simulink model "Hybrid_PV_Wind_System"  (R2018a)
settings: Solver=ode3  StartTime=0.0  StopTime=80  FixedStep=1e-4  RelTol=1e-3  EnableMultiTasking=on
InitFcn:
  | clear all ;
  | clc;
  | 
  | %%Wind System%%
  | 
  | %wind speed
  | Z_data=10;
  | Z_hub=85;
  | Z_0=0.03;
  | 
  | %Turbine
  | R_=45;
  | G=100;
  | lambda_opt=7.07;
  | Rho=1.225;
  | J=254;
  | f=0.01;
  | 
  | %RL filter;
  | 
  | fs=10000;
  | fe=50;
  | Ws=2*pi*fe;
  | Pres=3e6;
  | L=0.75e-3;
  | R=0.075;
  | c=38e-3;
  | 
  | %Commande CCR;
  | 
  | Id_=0;
  | Vdc_=1200;
  | %Vq_=0;
  | tr=0.001;
  | kp=3*L/tr;
  | ki=3*R/tr;
  | 
  | %CCM Commande;
  | 
  | p=2;
  | Tr=0.02;
  | Lfs=121e-6;
  | Lfr=57.3e-6;
  | Lm=12.12e-3;
  | m=1;
  | Ls=Lfs+Lm;
  | Lr=Lfr+m*Lm;
  | sigma=1-(m*Lm)^2/(Ls*Lr);
  | Rr=3.82e-3;
  | Rs=2.97e-3;
  | kpr=3*sigma*Lr/Tr;
  | kir=3*Rr/Tr;
  | Qs_ref=0;
  | 
  | %%PV SYSTEM%%
  | 
  | % T_cellule;
  | NOCT=45;
  | 
  | %PV module;
  | Ki=5e-4;
  | q=1.6e-19;
  | K=1.38e-23;
  | n=1.3;
  | Eg0=1.12;
  | Rs=.1;
  | Rp=515;
  | Tn=298.15;
  | Gn=1000;
  | Voc=46.5;
  | Isc=9.68;
  | Ns=72;
  | 
  | % Boost converter;
  | dv=3.1;   %53.85;
  | di=0.16;  %0.2053;
  | F=10000;
  | T=1/F;
  | %Vs=398;
  | Vab=690;         %sqrt(3)*Vs;
  | Vdc=1200;       %2*sqrt(2)*Vab/sqrt(3);
  | Vpv=303.2;
  | a=1-Vpv/Vdc;
  | Pn=350*40;
  | r=Vdc*Vdc/Pn;
  | l=0.5*Vpv*a*T/di;              %80e-3;
  | C=0.5*Vdc*a*T/(dv*r);       % 10e-6;
  | 
  | 
  | %Control PWM
  | Vgq=690/sqrt(3);
  | Fs=5000;
  | Ig=2*Pn/(3*690/sqrt(3)*sqrt(2));
  | dIg=0.05*Ig;
  | L1=690/(6*sqrt(2)*Fs*dIg);
  | R1=0.01;
  | 
  | 
  | tr1=1e-5;
  | Tau=tr1/3;
  | ki1=R1/Tau/Vgq;
  | kp1=L1/Tau/Vgq;
undefined symbols (not defined in the file): sigbuilder_block
libraries: powerlib_meascontrol x20, simulink x10
(part 1 of 2)
settings Model: Creator=PC  LastModifiedBy=yassine
settings OptimizationCC: LifeSpan=inf
settings DebuggingCC: SFUnexpectedBacktrackingDiag=warning  SFNoUnconditionalDefaultTransitionDiag=warning
settings CodeAppCC: StateflowObjectComments=on
settings GRTTargetCC: TargetLangStandard=C89/C90 (ANSI)
settings ConfigComp: CovMetricSettings=dw  CovSaveCumulativeToWorkspaceVar=on  CovSaveSingleToWorkspaceVar=on  CovExternalEMLEnable=off

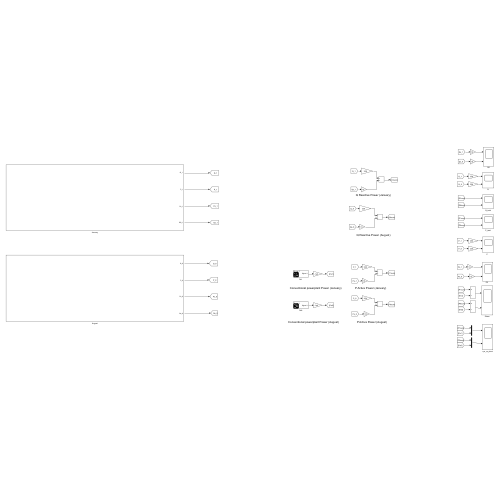
[thumbnail: Simulink's stored preview of the top-level diagram]
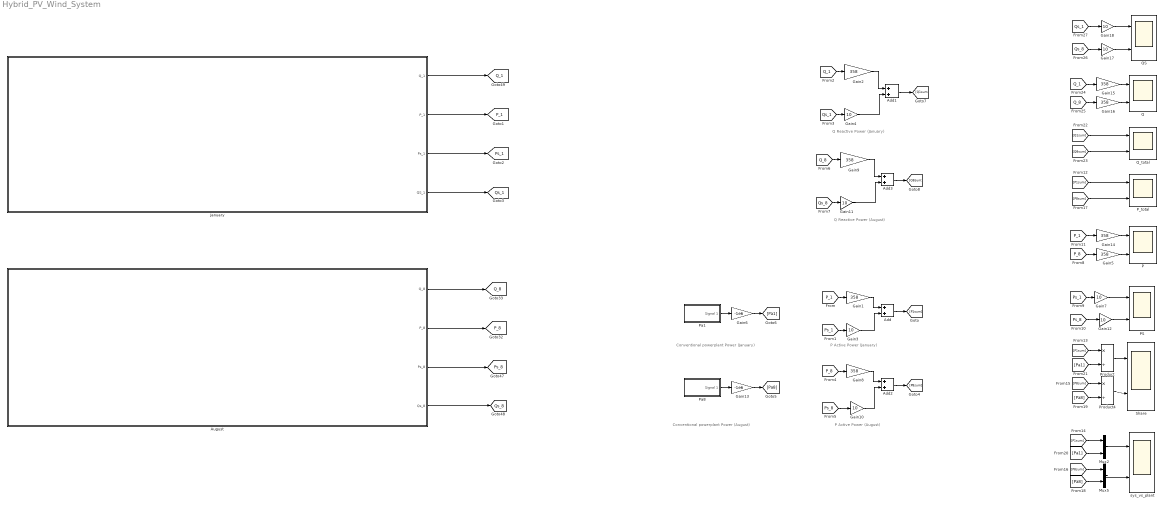
== system Hybrid_PV_Wind_System ==
  note: Conventional powerplant Power (January)
  note: Q Reactive Power (January)
  note: Q Reactive Power (August)
  note: P Active Power (January)
  note: P Active Power (August)
  note: Conventional powerplant Power (August)
  Add{,1..3} (4 alike) : Sum
  August : Subsystem
  Gain{1..2,5,8..9,14..16} (8 alike) : Gain  Gain=358
  Gain{3..4,7,10..12,17..18} (8 alike) : Gain  Gain=10
  Gain13 : Gain  Gain=-1e6
  Gain6 : Gain  Gain=-1e6
  January : Subsystem
  Mux2 : Mux  Inputs=2
  Mux5 : Mux  Inputs=2
  "P    " : Scope  NumInputPorts=2
  "PS   " : Scope  NumInputPorts=2
  P_total : Scope  NumInputPorts=2
  Pa1 : Subsystem  Tag=STV Subsys  LoadFcn=sigbuilder_block('load');  StartFcn=sigbuilder_block('start');  StopFcn=sigbuilder_block('stop');  ClipboardFcn=sigbuilder_block('clipboard');  mask(Sigbuilder block){tuvar=[0:10]}
      mask help: Simulink:masks:SigbuilderBlock_MD
      mask init:
      | if ~strcmp(get_param(bdroot(gcbh),'SimulationStatus'),'stopped') tuvar = sigbuilder_block('maskInit'); end
      settings: CopyFcn=sigbuilder_block('copy');  DeleteFcn=sigbuilder_block('delete');  ModelCloseFcn=sigbuilder_block('modelClose');  PreSaveFcn=sigbuilder_block('preSave');  PauseFcn=sigbuilder_block('pause');  ContinueFcn=sigbuilder_block('continue');  NameChangeFcn=sigbuilder_block('namechange');  OpenFcn=sigbuilder_block('open',[0 30 1920 992.25 ]);  CloseFcn=sigbuilder_block('close');
      mask Display: plot(0, 0, 100, 100,[2, 2, 32, 32, 2], [68, 8, 8, 68, 68],[32, 2], [38, 38], [32, 19, 2],[53, 60, 44], [32, 17, 17, 2],[16, 16, 31, 31]);txt = getActiveGroup(gcbh);text(2, 100, txt,'verticalAlignment', 'top');
  Pa8 : Subsystem  Tag=STV Subsys  LoadFcn=sigbuilder_block('load');  StartFcn=sigbuilder_block('start');  StopFcn=sigbuilder_block('stop');  ClipboardFcn=sigbuilder_block('clipboard');  mask(Sigbuilder block){tuvar=[0:10]}
      mask help: Simulink:masks:SigbuilderBlock_MD
      mask init:
      | if ~strcmp(get_param(bdroot(gcbh),'SimulationStatus'),'stopped') tuvar = sigbuilder_block('maskInit'); end
      settings: CopyFcn=sigbuilder_block('copy');  DeleteFcn=sigbuilder_block('delete');  ModelCloseFcn=sigbuilder_block('modelClose');  PreSaveFcn=sigbuilder_block('preSave');  PauseFcn=sigbuilder_block('pause');  ContinueFcn=sigbuilder_block('continue');  NameChangeFcn=sigbuilder_block('namechange');  OpenFcn=sigbuilder_block('open',[399 79.2 550.8 400.2 ]);  CloseFcn=sigbuilder_block('close');
      mask Display: plot(0, 0, 100, 100,[2, 2, 32, 32, 2], [68, 8, 8, 68, 68],[32, 2], [38, 38], [32, 19, 2],[53, 60, 44], [32, 17, 17, 2],[16, 16, 31, 31]);txt = getActiveGroup(gcbh);text(2, 100, txt,'verticalAlignment', 'top');
  Product : Product  Inputs=*/
  Product4 : Product  Inputs=*/
  Q : Scope  NumInputPorts=2
  QS : Scope  NumInputPorts=2
  Q_total : Scope  NumInputPorts=2
  Share : Scope  NumInputPorts=2
  sys_vs_plant : Scope  NumInputPorts=2
  tag scope: P_1=global, P_8=global, Ps_1=global, Ps_8=global, Q_1=global, Q_8=global, Qs_1=global, Qs_8=global
  wires:
  Gain4/1 -> Add1/2
  Gain11/1 -> Add3/2
  [Q_8] -> Gain9/1
  Add3/1 -> [Q8sum]
  Gain2/1 -> Add1/1
  Gain9/1 -> Add3/1
  [Qs_1] -> Gain4/1
  [Qs_8] -> Gain11/1
  [Q_1] -> Gain2/1
  Gain3/1 -> Add/2
  Mux2/1 -> sys_vs_plant/1
  Gain10/1 -> Add2/2
  [Ps_8] -> Gain10/1
  Product4/1 -> Share/2
  Mux5/1 -> sys_vs_plant/2
  [P_8] -> Gain8/1
  Gain8/1 -> Add2/1
  Pa1/1(Signal 1) -> Gain6/1
  [Ps_1] -> Gain3/1
  Add/1 -> [P1sum]
  [Pa1] -> Mux2/2
  [P_1] -> Gain1/1
  Pa8/1(Signal 1) -> Gain13/1
  [P8sum] -> Product4/1
  [Pa8] -> Mux5/2
  Product/1 -> Share/1
  Gain1/1 -> Add/1
  August/1(Q_8) -> [Q_8]
  August/2(P_8) -> [P_8]
  August/3(Ps_8) -> [Ps_8]
  August/4(Qs_8) -> [Qs_8]
  January/1("Q_1 ") -> [Q_1]
  January/2(P_1) -> [P_1]
  January/3(Ps_1) -> [Ps_1]
  January/4(QS_1) -> [Qs_1]
  [P_8] -> Gain5/1
  Gain5/1 -> "P    "/2
  [Ps_1] -> Gain7/1
  Gain7/1 -> "PS   "/1
  [Ps_8] -> Gain12/1
  Gain12/1 -> "PS   "/2
  [P_1] -> Gain14/1
  Gain14/1 -> "P    "/1
  [P1sum] -> P_total/1
  [P1sum] -> Product/1
  [P1sum] -> Mux2/1
  Add2/1 -> [P8sum]
  [P8sum] -> Mux5/1
  [P8sum] -> P_total/2
  Gain13/1 -> [Pa8]
  [Pa8] -> Product4/2
  Gain6/1 -> [Pa1]
  [Pa1] -> Product/2
  [Q1sum] -> Q_total/1
  [Q8sum] -> Q_total/2
  Add1/1 -> [Q1sum]
  Gain15/1 -> Q/1
  [Q_1] -> Gain15/1
  [Q_8] -> Gain16/1
  Gain16/1 -> Q/2
  Gain18/1 -> QS/1
  [Qs_8] -> Gain17/1
  Gain17/1 -> QS/2
  [Qs_1] -> Gain18/1

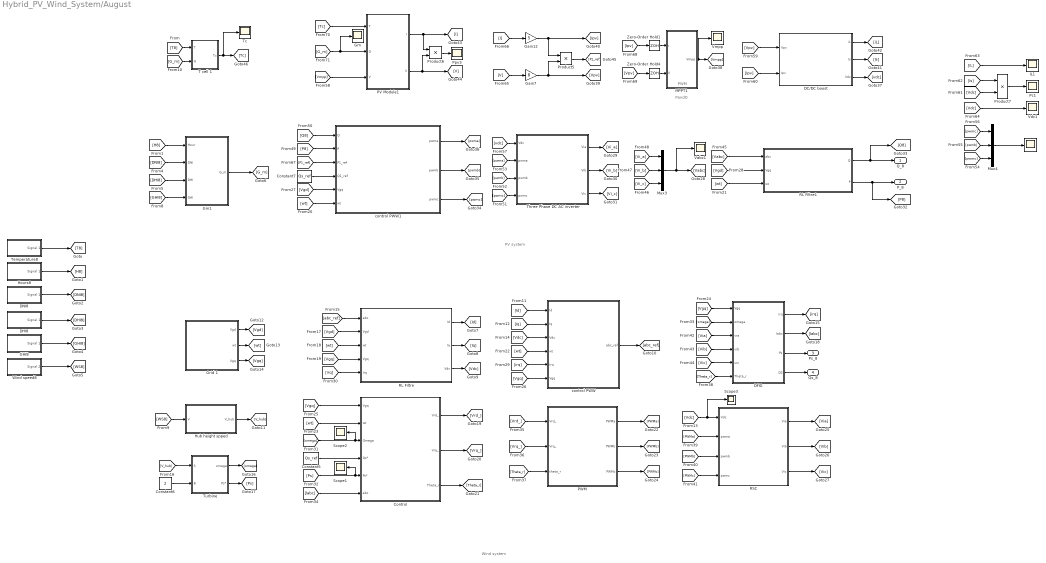
== system Hybrid_PV_Wind_System/August ==
  note: Wind system
  note: PWM
  note: PandO
  note: PV system
  " " : Scope
  Constant5 : Constant  Value=Qs_ref
  Constant6 : Constant  Value=2
  Constant7 : Constant  Value=Qs_ref
  Control : Subsystem
  DC/DC boost : Subsystem
  "DFIG " : Subsystem
  DHI8 : Subsystem  Tag=STV Subsys  LoadFcn=sigbuilder_block('load');  StartFcn=sigbuilder_block('start');  StopFcn=sigbuilder_block('stop');  ClipboardFcn=sigbuilder_block('clipboard');  mask(Sigbuilder block){tuvar=[0:10]}
      mask help: Simulink:masks:SigbuilderBlock_MD
      mask init:
      | if ~strcmp(get_param(bdroot(gcbh),'SimulationStatus'),'stopped') tuvar = sigbuilder_block('maskInit'); end
      settings: CopyFcn=sigbuilder_block('copy');  DeleteFcn=sigbuilder_block('delete');  ModelCloseFcn=sigbuilder_block('modelClose');  PreSaveFcn=sigbuilder_block('preSave');  PauseFcn=sigbuilder_block('pause');  ContinueFcn=sigbuilder_block('continue');  NameChangeFcn=sigbuilder_block('namechange');  OpenFcn=sigbuilder_block('open',[303.6 90.6 550.8 400.2 ]);  CloseFcn=sigbuilder_block('close');
      mask Display: plot(0, 0, 100, 100,[2, 2, 32, 32, 2], [68, 8, 8, 68, 68],[32, 2], [38, 38], [32, 19, 2],[53, 60, 44], [32, 17, 17, 2],[16, 16, 31, 31]);txt = getActiveGroup(gcbh);text(2, 100, txt,'verticalAlignment', 'top');
  DNI8 : Subsystem  Tag=STV Subsys  LoadFcn=sigbuilder_block('load');  StartFcn=sigbuilder_block('start');  StopFcn=sigbuilder_block('stop');  ClipboardFcn=sigbuilder_block('clipboard');  mask(Sigbuilder block){tuvar=[0:10]}
      mask help: Simulink:masks:SigbuilderBlock_MD
      mask init:
      | if ~strcmp(get_param(bdroot(gcbh),'SimulationStatus'),'stopped') tuvar = sigbuilder_block('maskInit'); end
      settings: CopyFcn=sigbuilder_block('copy');  DeleteFcn=sigbuilder_block('delete');  ModelCloseFcn=sigbuilder_block('modelClose');  PreSaveFcn=sigbuilder_block('preSave');  PauseFcn=sigbuilder_block('pause');  ContinueFcn=sigbuilder_block('continue');  NameChangeFcn=sigbuilder_block('namechange');  OpenFcn=sigbuilder_block('open',[446.4 127.8 550.8 400.2 ]);  CloseFcn=sigbuilder_block('close');
      mask Display: plot(0, 0, 100, 100,[2, 2, 32, 32, 2], [68, 8, 8, 68, 68],[32, 2], [38, 38], [32, 19, 2],[53, 60, 44], [32, 17, 17, 2],[16, 16, 31, 31]);txt = getActiveGroup(gcbh);text(2, 100, txt,'verticalAlignment', 'top');
  GHI8 : Subsystem  Tag=STV Subsys  LoadFcn=sigbuilder_block('load');  StartFcn=sigbuilder_block('start');  StopFcn=sigbuilder_block('stop');  ClipboardFcn=sigbuilder_block('clipboard');  mask(Sigbuilder block){tuvar=[0:10]}
      mask help: Simulink:masks:SigbuilderBlock_MD
      mask init:
      | if ~strcmp(get_param(bdroot(gcbh),'SimulationStatus'),'stopped') tuvar = sigbuilder_block('maskInit'); end
      settings: CopyFcn=sigbuilder_block('copy');  DeleteFcn=sigbuilder_block('delete');  ModelCloseFcn=sigbuilder_block('modelClose');  PreSaveFcn=sigbuilder_block('preSave');  PauseFcn=sigbuilder_block('pause');  ContinueFcn=sigbuilder_block('continue');  NameChangeFcn=sigbuilder_block('namechange');  OpenFcn=sigbuilder_block('open',[437.6 199.2 550.4 400 ]);  CloseFcn=sigbuilder_block('close');
      mask Display: plot(0, 0, 100, 100,[2, 2, 32, 32, 2], [68, 8, 8, 68, 68],[32, 2], [38, 38], [32, 19, 2],[53, 60, 44], [32, 17, 17, 2],[16, 16, 31, 31]);txt = getActiveGroup(gcbh);text(2, 100, txt,'verticalAlignment', 'top');
  Gain12 : Gain  Gain=5
  Gain7 : Gain  Gain=8
  "Gm  " : Scope
  Gm1 : Subsystem
  Grid 1 : Subsystem
  Hours8 : Subsystem  Tag=STV Subsys  LoadFcn=sigbuilder_block('load');  StartFcn=sigbuilder_block('start');  StopFcn=sigbuilder_block('stop');  ClipboardFcn=sigbuilder_block('clipboard');  mask(Sigbuilder block){tuvar=[0:10]}
      mask help: Simulink:masks:SigbuilderBlock_MD
      mask init:
      | if ~strcmp(get_param(bdroot(gcbh),'SimulationStatus'),'stopped') tuvar = sigbuilder_block('maskInit'); end
      settings: CopyFcn=sigbuilder_block('copy');  DeleteFcn=sigbuilder_block('delete');  ModelCloseFcn=sigbuilder_block('modelClose');  PreSaveFcn=sigbuilder_block('preSave');  PauseFcn=sigbuilder_block('pause');  ContinueFcn=sigbuilder_block('continue');  NameChangeFcn=sigbuilder_block('namechange');  OpenFcn=sigbuilder_block('open',[446.4 139.2 550.8 400.2 ]);  CloseFcn=sigbuilder_block('close');
      mask Display: plot(0, 0, 100, 100,[2, 2, 32, 32, 2], [68, 8, 8, 68, 68],[32, 2], [38, 38], [32, 19, 2],[53, 60, 44], [32, 17, 17, 2],[16, 16, 31, 31]);txt = getActiveGroup(gcbh);text(2, 100, txt,'verticalAlignment', 'top');
  Hub height spped : Subsystem
  IL1 : Scope
  MPPT1 : Subsystem
  Mux3 : Mux  Inputs=3
  Mux4 : Mux  Inputs=3
  PV Module1 : Subsystem
  PWM : Subsystem
  Pc1 : Scope
  Ppv3 : Scope
  Product5 : Product
  Product6 : Product
  Product7 : Product
  RL Filtre : Subsystem
  RL Filtre1 : Subsystem
  RSC : Subsystem
  Scope1 : Scope
  Scope2 : Scope
  Scope3 : Scope
  T cell 1 : Subsystem
  Tc : Scope
  Temperature8 : Subsystem  Tag=STV Subsys  LoadFcn=sigbuilder_block('load');  StartFcn=sigbuilder_block('start');  StopFcn=sigbuilder_block('stop');  ClipboardFcn=sigbuilder_block('clipboard');  mask(Sigbuilder block){tuvar=[0:10]}
      mask help: Simulink:masks:SigbuilderBlock_MD
      mask init:
      | if ~strcmp(get_param(bdroot(gcbh),'SimulationStatus'),'stopped') tuvar = sigbuilder_block('maskInit'); end
      settings: CopyFcn=sigbuilder_block('copy');  DeleteFcn=sigbuilder_block('delete');  ModelCloseFcn=sigbuilder_block('modelClose');  PreSaveFcn=sigbuilder_block('preSave');  PauseFcn=sigbuilder_block('pause');  ContinueFcn=sigbuilder_block('continue');  NameChangeFcn=sigbuilder_block('namechange');  OpenFcn=sigbuilder_block('open',[211.2 117.6 550.8 400.2 ]);  CloseFcn=sigbuilder_block('close');
      mask Display: plot(0, 0, 100, 100,[2, 2, 32, 32, 2], [68, 8, 8, 68, 68],[32, 2], [38, 38], [32, 19, 2],[53, 60, 44], [32, 17, 17, 2],[16, 16, 31, 31]);txt = getActiveGroup(gcbh);text(2, 100, txt,'verticalAlignment', 'top');
  Three Phase DC AC inverter : Subsystem
  Turbine : Subsystem
  Vabc1 : Scope
  Vdc1 : Scope
  Vmpp : Scope
  Wind speed8 : Subsystem  Tag=STV Subsys  LoadFcn=sigbuilder_block('load');  StartFcn=sigbuilder_block('start');  StopFcn=sigbuilder_block('stop');  ClipboardFcn=sigbuilder_block('clipboard');  mask(Sigbuilder block){tuvar=[0:10]}
      mask help: Simulink:masks:SigbuilderBlock_MD
      mask init:
      | if ~strcmp(get_param(bdroot(gcbh),'SimulationStatus'),'stopped') tuvar = sigbuilder_block('maskInit'); end
      settings: CopyFcn=sigbuilder_block('copy');  DeleteFcn=sigbuilder_block('delete');  ModelCloseFcn=sigbuilder_block('modelClose');  PreSaveFcn=sigbuilder_block('preSave');  PauseFcn=sigbuilder_block('pause');  ContinueFcn=sigbuilder_block('continue');  NameChangeFcn=sigbuilder_block('namechange');  OpenFcn=sigbuilder_block('open',[363 165 550.8 400.2 ]);  CloseFcn=sigbuilder_block('close');
      mask Display: plot(0, 0, 100, 100,[2, 2, 32, 32, 2], [68, 8, 8, 68, 68],[32, 2], [38, 38], [32, 19, 2],[53, 60, 44], [32, 17, 17, 2],[16, 16, 31, 31]);txt = getActiveGroup(gcbh);text(2, 100, txt,'verticalAlignment', 'top');
  Zero-Order Hold1 : ZeroOrderHold  SampleTime=1e-4
  Zero-Order Hold4 : ZeroOrderHold  SampleTime=1e-4
  "control PWW " : Subsystem
  control PWW1 : Subsystem
  Q_8 : Outport
  P_8 : Outport  Port=2
  Ps_8 : Outport  Port=3
  Qs_8 : Outport  Port=4
  wires:
  [Vrq_] -> PWM/2(Vrq_)
  [Via] -> "DFIG "/3(vra)
  [Vdc] -> Scope3/1, RSC/1(Vdc)
  [Vgd] -> RL Filtre/2(Vgd)
  Gain7/1 -> [Vpv], Product5/2
  DC/DC boost/3(Vdc) -> [vdc]
  [wt] -> RL Filtre/3(wt)
  [Vib] -> "DFIG "/4(vrb)
  [PWMb] -> RSC/3(pwmb)
  [T8] -> T cell 1/1(T)
  [Tc] -> PV Module1/1(T)
  [PWMa] -> RSC/2(pwma)
  [Vrd_] -> PWM/1(Vrd_)
  [Vgq] -> RL Filtre/4(Vgq)
  [PWMc] -> RSC/4(pwmc)
  Product6/1 -> Ppv3/1
  Mux4/1 -> " "/1
  [omega] -> Scope2/1, Control/3(Omega)
  [Theta_r] -> PWM/3(theta_r)
  [V_hub] -> Turbine/1(S)
  [Ps] -> Control/5(Ps*), Scope1/1
  Mux3/1 -> [Vabc], Vabc1/1
  Zero-Order Hold1/1 -> MPPT1/1(I)
  Constant7/1 -> control PWW1/4(Q1_ref)
  RL Filtre1/2(P) -> [P8], P_8/1
  [iL] -> IL1/1
  Product7/1 -> Pc1/1
  Gain12/1 -> [Ipv], Product5/1
  [DNI8] -> Gm1/2(DNI)
  [Vic] -> "DFIG "/5(vrc)
  Product5/1 -> [P1_ref]
  RL Filtre1/1("Q ") -> [Q8], Q_8/1
  Constant6/1 -> Turbine/2(B)
  [WS8] -> Hub height spped/1(V)
  [H8] -> Gm1/1(Hour)
  [DHI8] -> Gm1/3(DHI)
  [GHI8] -> Gm1/4(GHI)
  Zero-Order Hold4/1 -> MPPT1/2(V)
  Constant5/1 -> Control/4(Qs*)
  DNI8/1(Signal 1) -> [DNI8]
  DHI8/1(Signal 1) -> [DHI8]
  GHI8/1(Signal 1) -> [GHI8]
  Temperature8/1(Signal 1) -> [T8]
  Hours8/1(Signal 1) -> [H8]
  Wind speed8/1(Signal 2) -> [WS8]
  Gm1/1(G_m) -> [G_m]
  RL Filtre/1(Id) -> [Id]
  RL Filtre/2(Iq) -> [Iq]
  RL Filtre/3(Vdc) -> [Vdc]
  [Id] -> "control PWW "/1(Id)
  [Iq] -> "control PWW "/2(Iq)
  [Vdc] -> "control PWW "/3(Vdc)
  "control PWW "/1(abc_ref) -> [abc_ref]
  [abc_ref] -> RL Filtre/1(abc)
  Hub height spped/1(V_hub) -> [V_hub]
  Grid 1/1(Vgd) -> [Vgd]
  Grid 1/2(wt) -> [wt]
  Grid 1/3(Vgq) -> [Vgq]
  [wt] -> control PWW1/6(wt)
  [wt] -> RL Filtre1/3(wt)
  [wt] -> "control PWW "/4(wt)
  [wt] -> Control/2(wt)
  [Vgq] -> "DFIG "/1(Vgq)
  [Vgq] -> Control/1(Vgq)
  [Vgq] -> "control PWW "/6(Vgq)
  [Vgd] -> control PWW1/5(Vgq)
  [Vgd] -> RL Filtre1/2(Vgq)
  "DFIG "/1(irq) -> [irq]
  [irq] -> "control PWW "/5(Irq)
  [irq] -> RL Filtre/5(Irq)
  Turbine/1(omega) -> [omega]
  Turbine/2(Ps*) -> [Ps]
  [omega] -> "DFIG "/2(omega)
  "DFIG "/2(Iabc) -> [labc]
  [labc] -> Control/6(abc)
  Control/1(Vrd_) -> [Vrd_]
  Control/2(Vrq_) -> [Vrq_]
  Control/3(Theta_r) -> [Theta_r]
  [Theta_r] -> "DFIG "/6(Theta_r)
  PWM/1(PWMa) -> [PWMa]
  PWM/2(PWMb) -> [PWMb]
  PWM/3(PWMc) -> [PWMc]
  RSC/1(Via) -> [Via]
  RSC/2(Vib) -> [Vib]
  RSC/3(Vic) -> [Vic]
  [Vabc] -> RL Filtre1/1(abc)
  Three Phase DC AC inverter/1(Via) -> [Vi_a]
  Three Phase DC AC inverter/2(Vib) -> [Vi_b]
  Three Phase DC AC inverter/3(Vic) -> [Vi_c]
  [Vi_c] -> Mux3/3
  [Vi_b] -> Mux3/2
  [Vi_a] -> Mux3/1
  [P8] -> control PWW1/2(P)
  [Q8] -> control PWW1/1("Q ")
  control PWW1/3(pwmc) -> [pwmc]
  [pwmc] -> Three Phase DC AC inverter/4(pwmc)
  control PWW1/2(pwmb) -> [pwmb]
  [pwmb] -> Three Phase DC AC inverter/3(pwmb)
  control PWW1/1(pwma) -> [pwma]
  [pwma] -> Three Phase DC AC inverter/2(pwma)
  [pwmc] -> Mux4/3
  [pwmb] -> Mux4/2
  [pwmc] -> Mux4/1
  [vdc] -> Three Phase DC AC inverter/1(Vdc)
  MPPT1/1(Vmpp) -> Vmpp/1, [Vmpp]
  [Vmpp] -> PV Module1/3("V ")
  [Vpv] -> DC/DC boost/1(Vpv)
  [Ipv] -> DC/DC boost/2(Ipv)
  [Vdc] -> Product7/2
  DC/DC boost/2(Is) -> [Is]
  [Is] -> Product7/1
  DC/DC boost/1(iL) -> [iL]
  [Vdc] -> Vdc1/1
  [I] -> Gain12/1
  PV Module1/1(I) -> Product6/1, [I]
  [V] -> Gain7/1
  PV Module1/2(V) -> [V], Product6/2
  [P1_ref] -> control PWW1/3(P1_ref)
  [Vpv] -> Zero-Order Hold4/1
  [Ipv] -> Zero-Order Hold1/1
  T cell 1/1(Tc) -> Tc/1, [Tc]
  [G_m] -> T cell 1/2(G)
  [G_m] -> "Gm  "/1, PV Module1/2(G)
  "DFIG "/4(QS) -> Qs_8/1
  "DFIG "/3(Ps) -> Ps_8/1

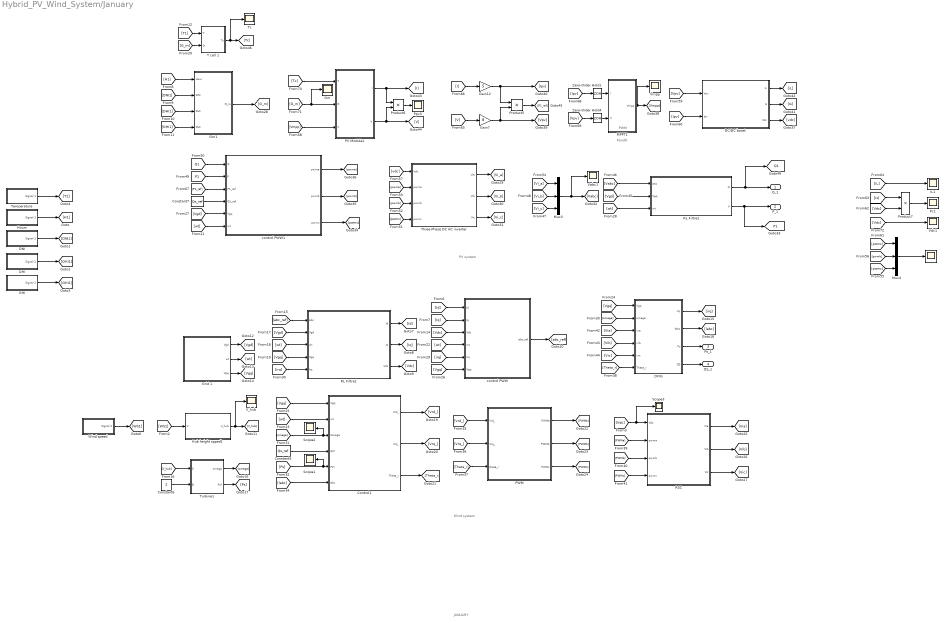
== system Hybrid_PV_Wind_System/January ==
  note: JANUARY
  note: PandO
  note: PWM
  note: PV system
  note: Wind system
  " " : Scope
  Constant5 : Constant  Value=Qs_ref
  Constant6 : Constant  Value=2
  Constant7 : Constant  Value=Qs_ref
  Control1 : Subsystem
  DC/DC boost : Subsystem
  "DFIG " : Subsystem
  DHI : Subsystem  Tag=STV Subsys  LoadFcn=sigbuilder_block('load');  StartFcn=sigbuilder_block('start');  StopFcn=sigbuilder_block('stop');  ClipboardFcn=sigbuilder_block('clipboard');  mask(Sigbuilder block){tuvar=[0:10]}
      mask help: Simulink:masks:SigbuilderBlock_MD
      mask init:
      | if ~strcmp(get_param(bdroot(gcbh),'SimulationStatus'),'stopped') tuvar = sigbuilder_block('maskInit'); end
      settings: CopyFcn=sigbuilder_block('copy');  DeleteFcn=sigbuilder_block('delete');  ModelCloseFcn=sigbuilder_block('modelClose');  PreSaveFcn=sigbuilder_block('preSave');  PauseFcn=sigbuilder_block('pause');  ContinueFcn=sigbuilder_block('continue');  NameChangeFcn=sigbuilder_block('namechange');  OpenFcn=sigbuilder_block('open',[303.6 90.6 550.8 400.2 ]);  CloseFcn=sigbuilder_block('close');
      mask Display: plot(0, 0, 100, 100,[2, 2, 32, 32, 2], [68, 8, 8, 68, 68],[32, 2], [38, 38], [32, 19, 2],[53, 60, 44], [32, 17, 17, 2],[16, 16, 31, 31]);txt = getActiveGroup(gcbh);text(2, 100, txt,'verticalAlignment', 'top');
  DNI : Subsystem  Tag=STV Subsys  LoadFcn=sigbuilder_block('load');  StartFcn=sigbuilder_block('start');  StopFcn=sigbuilder_block('stop');  ClipboardFcn=sigbuilder_block('clipboard');  mask(Sigbuilder block){tuvar=[0:10]}
      mask help: Simulink:masks:SigbuilderBlock_MD
      mask init:
      | if ~strcmp(get_param(bdroot(gcbh),'SimulationStatus'),'stopped') tuvar = sigbuilder_block('maskInit'); end
      settings: CopyFcn=sigbuilder_block('copy');  DeleteFcn=sigbuilder_block('delete');  ModelCloseFcn=sigbuilder_block('modelClose');  PreSaveFcn=sigbuilder_block('preSave');  PauseFcn=sigbuilder_block('pause');  ContinueFcn=sigbuilder_block('continue');  NameChangeFcn=sigbuilder_block('namechange');  OpenFcn=sigbuilder_block('open',[446.4 127.8 550.8 400.2 ]);  CloseFcn=sigbuilder_block('close');
      mask Display: plot(0, 0, 100, 100,[2, 2, 32, 32, 2], [68, 8, 8, 68, 68],[32, 2], [38, 38], [32, 19, 2],[53, 60, 44], [32, 17, 17, 2],[16, 16, 31, 31]);txt = getActiveGroup(gcbh);text(2, 100, txt,'verticalAlignment', 'top');
  GHI : Subsystem  Tag=STV Subsys  LoadFcn=sigbuilder_block('load');  StartFcn=sigbuilder_block('start');  StopFcn=sigbuilder_block('stop');  ClipboardFcn=sigbuilder_block('clipboard');  mask(Sigbuilder block){tuvar=[0:10]}
      mask help: Simulink:masks:SigbuilderBlock_MD
      mask init:
      | if ~strcmp(get_param(bdroot(gcbh),'SimulationStatus'),'stopped') tuvar = sigbuilder_block('maskInit'); end
      settings: CopyFcn=sigbuilder_block('copy');  DeleteFcn=sigbuilder_block('delete');  ModelCloseFcn=sigbuilder_block('modelClose');  PreSaveFcn=sigbuilder_block('preSave');  PauseFcn=sigbuilder_block('pause');  ContinueFcn=sigbuilder_block('continue');  NameChangeFcn=sigbuilder_block('namechange');  OpenFcn=sigbuilder_block('open',[437.6 199.2 550.4 400 ]);  CloseFcn=sigbuilder_block('close');
      mask Display: plot(0, 0, 100, 100,[2, 2, 32, 32, 2], [68, 8, 8, 68, 68],[32, 2], [38, 38], [32, 19, 2],[53, 60, 44], [32, 17, 17, 2],[16, 16, 31, 31]);txt = getActiveGroup(gcbh);text(2, 100, txt,'verticalAlignment', 'top');
  Gain12 : Gain  Gain=5
  Gain7 : Gain  Gain=8
  "Gm  " : Scope
  Gm1 : Subsystem
  Grid 1 : Subsystem
  Hours : Subsystem  Tag=STV Subsys  LoadFcn=sigbuilder_block('load');  StartFcn=sigbuilder_block('start');  StopFcn=sigbuilder_block('stop');  ClipboardFcn=sigbuilder_block('clipboard');  mask(Sigbuilder block){tuvar=[0:10]}
      mask help: Simulink:masks:SigbuilderBlock_MD
      mask init:
      | if ~strcmp(get_param(bdroot(gcbh),'SimulationStatus'),'stopped') tuvar = sigbuilder_block('maskInit'); end
      settings: CopyFcn=sigbuilder_block('copy');  DeleteFcn=sigbuilder_block('delete');  ModelCloseFcn=sigbuilder_block('modelClose');  PreSaveFcn=sigbuilder_block('preSave');  PauseFcn=sigbuilder_block('pause');  ContinueFcn=sigbuilder_block('continue');  NameChangeFcn=sigbuilder_block('namechange');  OpenFcn=sigbuilder_block('open',[446.4 139.2 550.8 400.2 ]);  CloseFcn=sigbuilder_block('close');
      mask Display: plot(0, 0, 100, 100,[2, 2, 32, 32, 2], [68, 8, 8, 68, 68],[32, 2], [38, 38], [32, 19, 2],[53, 60, 44], [32, 17, 17, 2],[16, 16, 31, 31]);txt = getActiveGroup(gcbh);text(2, 100, txt,'verticalAlignment', 'top');
  Hub height spped1 : Subsystem
  IL1 : Scope
  MPPT1 : Subsystem
  Mux3 : Mux  Inputs=3
  Mux4 : Mux  Inputs=3
  PV Module1 : Subsystem
  PWM : Subsystem
  Pc1 : Scope
  Ppv3 : Scope
  Product5 : Product
  Product6 : Product
  Product7 : Product
  RL Filtre1 : Subsystem
  RL Filtre2 : Subsystem
  RSC : Subsystem
  Scope1 : Scope
  Scope2 : Scope
  Scope3 : Scope
  T cell 1 : Subsystem
  Tc : Scope
  Temperature : Subsystem  Tag=STV Subsys  LoadFcn=sigbuilder_block('load');  StartFcn=sigbuilder_block('start');  StopFcn=sigbuilder_block('stop');  ClipboardFcn=sigbuilder_block('clipboard');  mask(Sigbuilder block){tuvar=[0:10]}
      mask help: Simulink:masks:SigbuilderBlock_MD
      mask init:
      | if ~strcmp(get_param(bdroot(gcbh),'SimulationStatus'),'stopped') tuvar = sigbuilder_block('maskInit'); end
      settings: CopyFcn=sigbuilder_block('copy');  DeleteFcn=sigbuilder_block('delete');  ModelCloseFcn=sigbuilder_block('modelClose');  PreSaveFcn=sigbuilder_block('preSave');  PauseFcn=sigbuilder_block('pause');  ContinueFcn=sigbuilder_block('continue');  NameChangeFcn=sigbuilder_block('namechange');  OpenFcn=sigbuilder_block('open',[310.8 67.2 550.8 400.2 ]);  CloseFcn=sigbuilder_block('close');
      mask Display: plot(0, 0, 100, 100,[2, 2, 32, 32, 2], [68, 8, 8, 68, 68],[32, 2], [38, 38], [32, 19, 2],[53, 60, 44], [32, 17, 17, 2],[16, 16, 31, 31]);txt = getActiveGroup(gcbh);text(2, 100, txt,'verticalAlignment', 'top');
  Three Phase DC AC inverter : Subsystem
  Turbine1 : Subsystem
  V_hub : Scope
  Vabc1 : Scope
  Vdc1 : Scope
  Vmpp : Scope
  Wind speed : Subsystem  Tag=STV Subsys  LoadFcn=sigbuilder_block('load');  StartFcn=sigbuilder_block('start');  StopFcn=sigbuilder_block('stop');  ClipboardFcn=sigbuilder_block('clipboard');  mask(Sigbuilder block){tuvar=[0:10]}
      mask help: Simulink:masks:SigbuilderBlock_MD
      mask init:
      | if ~strcmp(get_param(bdroot(gcbh),'SimulationStatus'),'stopped') tuvar = sigbuilder_block('maskInit'); end
      settings: CopyFcn=sigbuilder_block('copy');  DeleteFcn=sigbuilder_block('delete');  ModelCloseFcn=sigbuilder_block('modelClose');  PreSaveFcn=sigbuilder_block('preSave');  PauseFcn=sigbuilder_block('pause');  ContinueFcn=sigbuilder_block('continue');  NameChangeFcn=sigbuilder_block('namechange');  OpenFcn=sigbuilder_block('open',[268.2 96 550.8 400.2 ]);  CloseFcn=sigbuilder_block('close');
      mask Display: plot(0, 0, 100, 100,[2, 2, 32, 32, 2], [68, 8, 8, 68, 68],[32, 2], [38, 38], [32, 19, 2],[53, 60, 44], [32, 17, 17, 2],[16, 16, 31, 31]);txt = getActiveGroup(gcbh);text(2, 100, txt,'verticalAlignment', 'top');
  Zero-Order Hold1 : ZeroOrderHold  SampleTime=1e-4
  Zero-Order Hold4 : ZeroOrderHold  SampleTime=1e-4
  "control PWW " : Subsystem
  control PWW1 : Subsystem
  "Q_1 " : Outport
  P_1 : Outport  Port=2
  Ps_1 : Outport  Port=3
  QS_1 : Outport  Port=4
  tag scope: P1=global, Q1=global
  wires:
  Hub height spped1/1(V_hub) -> [V_hub], V_hub/1
  Temperature/1(Signal 1) -> [T1]
  Wind speed/1(Signal 2) -> [WS1]
  DNI/1(Signal 1) -> [DNI1]
  DHI/1(Signal 1) -> [DHI1]
  GHI/1(Signal 1) -> [GHI1]
  Hours/1(Signal 1) -> [H1]
  Turbine1/1(omega) -> [omega]
  Turbine1/2(Ps*) -> [Ps]
  [WS1] -> Hub height spped1/1(V)
  Constant6/1 -> Turbine1/2(B)
  [V_hub] -> Turbine1/1(S)
  Control1/1(Vrd_) -> [Vrd_]
  [wt] -> Control1/2(wt)
  Control1/2(Vrq_) -> [Vrq_]
  [Vgq] -> Control1/1(Vgq)
  Control1/3(Theta_r) -> [Theta_r]
  Constant5/1 -> Control1/4(Qs*)
  [labc] -> Control1/6(abc)
  [omega] -> Scope2/1, Control1/3(Omega)
  [Ps] -> Control1/5(Ps*), Scope1/1
  PWM/2(PWMb) -> [PWMb]
  PWM/1(PWMa) -> [PWMa]
  [Theta_r] -> PWM/3(theta_r)
  PWM/3(PWMc) -> [PWMc]
  [Vrq_] -> PWM/2(Vrq_)
  [Vrd_] -> PWM/1(Vrd_)
  [PWMa] -> RSC/2(pwma)
  [Vdc] -> Scope3/1, RSC/1(Vdc)
  RSC/2(Vib) -> [Vib]
  [PWMc] -> RSC/4(pwmc)
  [PWMb] -> RSC/3(pwmb)
  RSC/3(Vic) -> [Vic]
  RSC/1(Via) -> [Via]
  "DFIG "/2(Iabc) -> [labc]
  [Theta_r] -> "DFIG "/6(Theta_r)
  [Vib] -> "DFIG "/4(vrb)
  "DFIG "/3(Ps) -> Ps_1/1
  "DFIG "/4(QS) -> QS_1/1
  [omega] -> "DFIG "/2(omega)
  [Vgq] -> "DFIG "/1(Vgq)
  [Vic] -> "DFIG "/5(vrc)
  [Via] -> "DFIG "/3(vra)
  "DFIG "/1(irq) -> [irq]
  Grid 1/1(Vgd) -> [Vgd]
  Grid 1/3(Vgq) -> [Vgq]
  Grid 1/2(wt) -> [wt]
  RL Filtre1/2(Iq) -> [Iq]
  [irq] -> RL Filtre1/5(Irq)
  RL Filtre1/3(Vdc) -> [Vdc]
  [abc_ref] -> RL Filtre1/1(abc)
  [Vgq] -> RL Filtre1/4(Vgq)
  [wt] -> RL Filtre1/3(wt)
  [Vgd] -> RL Filtre1/2(Vgd)
  RL Filtre1/1(Id) -> [Id]
  [Iq] -> "control PWW "/2(Iq)
  [irq] -> "control PWW "/5(Irq)
  [Vgq] -> "control PWW "/6(Vgq)
  "control PWW "/1(abc_ref) -> [abc_ref]
  [wt] -> "control PWW "/4(wt)
  [Id] -> "control PWW "/1(Id)
  [Vdc] -> "control PWW "/3(Vdc)
  [DHI1] -> Gm1/3(DHI)
  [H1] -> Gm1/1(Hour)
  [DNI1] -> Gm1/2(DNI)
  Gm1/1(G_m) -> [G_m]
  [GHI1] -> Gm1/4(GHI)
  [G_m] -> T cell 1/2(G)
  T cell 1/1(Tc) -> Tc/1, [Tc]
  [T1] -> T cell 1/1(T)
  PV Module1/1(I) -> Product6/1, [I]
  [G_m] -> "Gm  "/1, PV Module1/2(G)
  Product6/1 -> Ppv3/1
  [Vmpp] -> PV Module1/3("V ")
  [Tc] -> PV Module1/1(T)
  PV Module1/2(V) -> [V], Product6/2
  Constant7/1 -> control PWW1/4(Q1_ref)
  [P1_ref] -> control PWW1/3(P1_ref)
  [P1] -> control PWW1/2(P)
  control PWW1/3(pwmc) -> [pwmc]
  [Q1] -> control PWW1/1("Q ")
  [Vgd] -> control PWW1/5(Vgq)
  control PWW1/2(pwmb) -> [pwmb]
  [wt] -> control PWW1/6(wt)
  control PWW1/1(pwma) -> [pwma]
  Three Phase DC AC inverter/2(Vib) -> [Vi_b]
  [vdc] -> Three Phase DC AC inverter/1(Vdc)
  [pwma] -> Three Phase DC AC inverter/2(pwma)
  [pwmc] -> Three Phase DC AC inverter/4(pwmc)
  Three Phase DC AC inverter/3(Vic) -> [Vi_c]
  Three Phase DC AC inverter/1(Via) -> [Vi_a]
  [pwmb] -> Three Phase DC AC inverter/3(pwmb)
  [I] -> Gain12/1
  MPPT1/1(Vmpp) -> Vmpp/1, [Vmpp]
  [Vpv] -> Zero-Order Hold4/1
  Product5/1 -> [P1_ref]
  [Ipv] -> Zero-Order Hold1/1
  [V] -> Gain7/1
  Gain12/1 -> [Ipv], Product5/1
  Zero-Order Hold1/1 -> MPPT1/1(I)
  Zero-Order Hold4/1 -> MPPT1/2(V)
  Gain7/1 -> [Vpv], Product5/2
  [Vpv] -> DC/DC boost/1(Vpv)
  DC/DC boost/2(Is) -> [Is]
  [Ipv] -> DC/DC boost/2(Ipv)
  DC/DC boost/3(Vdc) -> [vdc]
  DC/DC boost/1(iL) -> [iL]
  [Vabc] -> RL Filtre2/1(abc)
  [Vi_c] -> Mux3/3
  [Vi_a] -> Mux3/1
  [Vi_b] -> Mux3/2
  [wt] -> RL Filtre2/3(wt)
  RL Filtre2/1("Q ") -> [Q1], "Q_1 "/1
  RL Filtre2/2(P) -> [P1], P_1/1
  Mux3/1 -> [Vabc], Vabc1/1
  [Vgd] -> RL Filtre2/2(Vgq)
  [iL] -> IL1/1
  [Vdc] -> Product7/2
  Mux4/1 -> " "/1
  [pwmb] -> Mux4/2
  [pwmc] -> Mux4/3
  [Vdc] -> Vdc1/1
  Product7/1 -> Pc1/1
  [Is] -> Product7/1
  [pwmc] -> Mux4/1

== system Hybrid_PV_Wind_System/Pa1 ==
  Demux : Demux  Tag=STV Demux  Outputs=1
      settings: DisplayOption=none
  FromWs : FromWorkspace  Tag=STV FromWs  VariableName=tuvar
      SigBuilderData=|
      | common.afterFinalStr = 'Extrapolate'
      | common.sampleTime = 0
      | dataSet.timeRange = [0 750]
      | dataSet.name = 'Group 1'
      | sbobj.Groups.Name = 'Group 1'
      | sbobj.Groups.Signals.Name = 'Signal 1'
      | sbobj.Groups.Signals.XData = [0 1 2 3 4 5 6 7 8 9 10 11 ... (745 elements, 1x745)]
      | sbobj.Groups.Signals.YData = [24.5 22.25 23 22 22 24 23.5 31.75 30.75 23.25 26.5 25 ... (745 elements, 1x745)]
      | sbobj.Groups.TimeRange = [0 750]
  Signal 1 : Outport  Tag=STV Outport
  wires:
  FromWs/1 -> Demux/1
  Demux/1 -> Signal 1/1

== system Hybrid_PV_Wind_System/Pa8 ==
  Demux : Demux  Tag=STV Demux  Outputs=1
      settings: DisplayOption=none
  FromWs : FromWorkspace  Tag=STV FromWs  VariableName=tuvar
      SigBuilderData=|
      | common.afterFinalStr = 'Extrapolate'
      | common.sampleTime = 0
      | dataSet.timeRange = [0 750]
      | dataSet.name = 'Group 1'
      | sbobj.Groups.Name = 'Group 1'
      | sbobj.Groups.Signals.Name = 'Signal 1'
      | sbobj.Groups.Signals.XData = [0 1 2 3 4 5 6 7 8 9 10 11 ... (745 elements, 1x745)]
      | sbobj.Groups.Signals.YData = [37.5 40.75 43.25 43.5 41.25 44 42 42 39 40.25 34.25 38.5 ... (745 elements, 1x745)]
      | sbobj.Groups.TimeRange = [0 750]
  Signal 1 : Outport  Tag=STV Outport
  wires:
  FromWs/1 -> Demux/1
  Demux/1 -> Signal 1/1

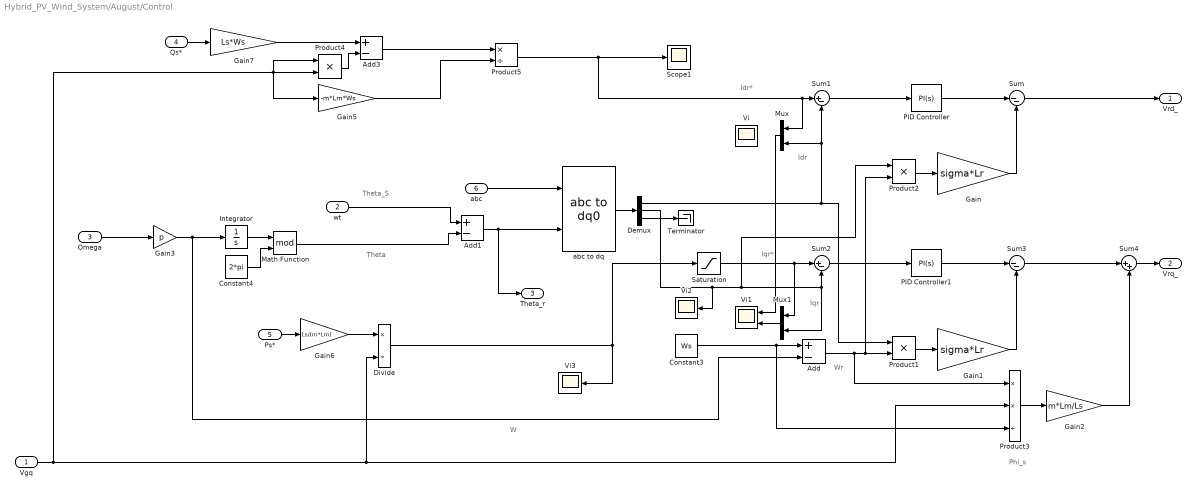
== system Hybrid_PV_Wind_System/August/Control ==
  note: Theta_S
  note: Theta
  note: W
  note: Wr
  note: Iqr
  note: Idr
  note: Phi_s
  note: Idr*
  note: Iqr*
  Vgq : Inport
  wt : Inport  Port=2
  Omega : Inport  Port=3
  Qs* : Inport  Port=4
  Ps* : Inport  Port=5
  abc : Inport  Port=6
  Add : Sum  Inputs=+-
  Add1 : Sum  Inputs=+-
  Add3 : Sum  Inputs=+-
  Constant3 : Constant  Value=Ws
  Constant4 : Constant  Value=2*pi
  Demux : Demux  Outputs=3
  Divide : Product  Inputs=*/
  Gain : Gain  Gain=sigma*Lr
  Gain1 : Gain  Gain=sigma*Lr
  Gain2 : Gain  Gain=m*Lm/Ls
  Gain3 : Gain  Gain=p
  Gain5 : Gain  Gain=-m*Lm*Ws
  Gain6 : Gain  Gain=Ls/(m*Lm)
  Gain7 : Gain  Gain=Ls*Ws
  Integrator : Integrator
  Math Function : Math  Operator=mod  SaturateOnIntegerOverflow=on
  Mux : Mux  Inputs=2
  Mux1 : Mux  Inputs=2
  PID Controller : simulink/Continuous/PID Controller  Controller=PI  Form=Parallel  TimeDomain=Continuous-time  SampleTime=-1  IntegratorMethod=Forward Euler  ControllerParametersSource=internal  P=kpr*62  I=kir*62  D=0  N=100  UseFilter=on  TunerSelectOption=Transfer Function Based (PID Tuner App)  InitialConditionSource=internal  InitialConditionForIntegrator=0  InitialConditionForFilter=0  DifferentiatorICPrevScaledInput=0  ExternalReset=none  TrackingMode=off  Kt=1  LimitOutput=off  UpperSaturationLimit=inf  LowerSaturationLimit=-inf  LinearizeAsGain=on  AntiWindupMode=none  Kb=1  POutMin=[]  POutMax=[]  IOutMin=[]  IOutMax=[]  DOutMin=[]  DOutMax=[]  NOutMin=[]  NOutMax=[]  SumOutMin=[]  SumOutMax=[]  SaturationOutMin=[]  SaturationOutMax=[]  PParamMin=[]  PParamMax=[]  IParamMin=[]  IParamMax=[]  DParamMin=[]  DParamMax=[]  NParamMin=[]  NParamMax=[]  KbParamMin=[]  KbParamMax=[]  KtParamMin=[]  KtParamMax=[]  KbOutMin=[]  KbOutMax=[]  KtOutMin=[]  KtOutMax=[]  IntegratorOutMin=[]  IntegratorOutMax=[]  FilterOutMin=[]  FilterOutMax=[]  SumI1OutMin=[]  SumI1OutMax=[]  SumI2OutMin=[]  SumI2OutMax=[]  SumI3OutMin=[]  SumI3OutMax=[]  SumDOutMin=[]  SumDOutMax=[]  DifferentiatorOutMin=[]  DifferentiatorOutMax=[]  FilterDiffOutCoefMin=[]  FilterDiffOutCoefMax=[]  ReciprocalOutMin=[]  ReciprocalOutMax=[]  SumDenOutMin=[]  SumDenOutMax=[]  SumNumOutMin=[]  SumNumOutMax=[]  DivideOutMin=[]  DivideOutMax=[]  IntegratorContinuousStateAttributes=''  IntegratorStateMustResolveToSignalObject=off  IntegratorRTWStateStorageClass=Auto  FilterContinuousStateAttributes=''  FilterStateMustResolveToSignalObject=off  FilterRTWStateStorageClass=Auto
  PID Controller1 : simulink/Continuous/PID Controller  Controller=PI  Form=Parallel  TimeDomain=Continuous-time  SampleTime=-1  IntegratorMethod=Forward Euler  ControllerParametersSource=internal  P=kpr*62  I=kir*62  D=0  N=100  UseFilter=on  TunerSelectOption=Transfer Function Based (PID Tuner App)  InitialConditionSource=internal  InitialConditionForIntegrator=0  InitialConditionForFilter=0  DifferentiatorICPrevScaledInput=0  ExternalReset=none  TrackingMode=off  Kt=1  LimitOutput=off  UpperSaturationLimit=inf  LowerSaturationLimit=-inf  LinearizeAsGain=on  AntiWindupMode=none  Kb=1  POutMin=[]  POutMax=[]  IOutMin=[]  IOutMax=[]  DOutMin=[]  DOutMax=[]  NOutMin=[]  NOutMax=[]  SumOutMin=[]  SumOutMax=[]  SaturationOutMin=[]  SaturationOutMax=[]  PParamMin=[]  PParamMax=[]  IParamMin=[]  IParamMax=[]  DParamMin=[]  DParamMax=[]  NParamMin=[]  NParamMax=[]  KbParamMin=[]  KbParamMax=[]  KtParamMin=[]  KtParamMax=[]  KbOutMin=[]  KbOutMax=[]  KtOutMin=[]  KtOutMax=[]  IntegratorOutMin=[]  IntegratorOutMax=[]  FilterOutMin=[]  FilterOutMax=[]  SumI1OutMin=[]  SumI1OutMax=[]  SumI2OutMin=[]  SumI2OutMax=[]  SumI3OutMin=[]  SumI3OutMax=[]  SumDOutMin=[]  SumDOutMax=[]  DifferentiatorOutMin=[]  DifferentiatorOutMax=[]  FilterDiffOutCoefMin=[]  FilterDiffOutCoefMax=[]  ReciprocalOutMin=[]  ReciprocalOutMax=[]  SumDenOutMin=[]  SumDenOutMax=[]  SumNumOutMin=[]  SumNumOutMax=[]  DivideOutMin=[]  DivideOutMax=[]  IntegratorContinuousStateAttributes=''  IntegratorStateMustResolveToSignalObject=off  IntegratorRTWStateStorageClass=Auto  FilterContinuousStateAttributes=''  FilterStateMustResolveToSignalObject=off  FilterRTWStateStorageClass=Auto
  Product1 : Product
  Product2 : Product
  Product3 : Product  Inputs=**/
  Product4 : Product  Inputs=**
  Product5 : Product  Inputs=*/
  Saturation : Saturate  UpperLimit=8e3  LowerLimit=-8e3
  Scope1 : Scope
  Sum : Sum  Inputs=|--
  Sum1 : Sum  Inputs=|+-
  Sum2 : Sum  Inputs=|+-
  Sum3 : Sum  Inputs=|--
  Sum4 : Sum  Inputs=|++
  Terminator : Terminator
  Vi : Scope
  Vi1 : Scope  NumInputPorts=2
  Vi2 : Scope
  Vi3 : Scope
  abc to dq : powerlib_meascontrol/Transformations/abc to dq0  Alignment=90 degrees behind phase A axis
  Vrd_ : Outport
  Vrq_ : Outport  Port=2
  Theta_r : Outport  Port=3
  wires:
  Sum2/1 -> PID Controller1/1
  Sum1/1 -> PID Controller/1
  Demux/2 -> Vi2/1, Mux1/2, Sum2/2, Product2/1
  PID Controller/1 -> Sum/1
  Gain/1 -> Sum/2
  Sum4/1 -> Vrq_/1
  PID Controller1/1 -> Sum3/1
  Demux/1 -> Sum1/2, Mux/2, Product1/1
  Gain2/1 -> Sum4/2
  Sum3/1 -> Sum4/1
  Sum/1 -> Vrd_/1
  Gain1/1 -> Sum3/2
  Constant3/1 -> Product3/3, Add/1
  Product1/1 -> Gain1/1
  Add/1 -> Product3/1, Product2/2, Product1/2
  Omega/1 -> Gain3/1
  Product2/1 -> Gain/1
  Product3/1 -> Gain2/1
  abc to dq/1 -> Demux/1
  Demux/3 -> Terminator/1
  abc/1 -> abc to dq/1
  wt/1 -> Add1/1
  Integrator/1 -> Math Function/1
  Constant4/1 -> Math Function/2
  Math Function/1 -> Add1/2
  Gain3/1 -> Integrator/1, Add/2
  Mux/1 -> Vi1/1
  Mux1/1 -> Vi1/2
  Add1/1 -> abc to dq/2, Theta_r/1
  Add3/1 -> Product5/1
  Vgq/1 -> Product3/2, Divide/2, Product4/1, Gain5/1, Product4/2
  Qs*/1 -> Gain7/1
  Gain5/1 -> Product5/2
  Product5/1 -> Sum1/1, Mux/1, Scope1/1
  Ps*/1 -> Gain6/1
  Gain6/1 -> Divide/1
  Gain7/1 -> Add3/1
  Product4/1 -> Add3/2
  Divide/1 -> Vi3/1, Saturation/1
  Saturation/1 -> Mux1/1, Sum2/1

== system Hybrid_PV_Wind_System/August/DC//DC boost ==
  Vpv : Inport
  Ipv : Inport  Port=2
  Add : Sum  Inputs=+-
  Gain : Gain  Gain=1/l
  Gain1 : Gain  Gain=1/l
  Gain2 : Gain  Gain=1/C
  Gain3 : Gain  Gain=1/(r*C)
  Integrator : Integrator
  Integrator1 : Integrator
  Product : Product
  Product1 : Product
  Product2 : Product  Inputs=*/
  Product4 : Product
  Sum : Sum  Inputs=|+-
  Sum1 : Sum  Inputs=|+-
  Sum2 : Sum  Inputs=|+-
  const : Constant
  const2 : Constant  Value=Vdc
  iL : Outport
  Is : Outport  Port=2
  Vdc : Outport  Port=3
  wires:
  Gain3/1 -> Sum2/2
  Integrator1/1 -> Vdc/1, Product/2, Gain3/1
  Sum2/1 -> Integrator1/1
  Product1/1 -> Gain2/1
  Product/1 -> Gain1/1
  Sum1/1 -> Integrator/1
  Gain1/1 -> Sum1/2
  Gain2/1 -> Sum2/1
  Gain/1 -> Sum1/1
  Add/1 -> Sum/2
  const/1 -> Add/1, Sum/1
  Vpv/1 -> Product2/1, Gain/1
  const2/1 -> Product2/2
  Product2/1 -> Add/2
  Sum/1 -> Product/1, Product4/1, Product1/1
  Integrator/1 -> iL/1, Product1/2
  Product4/1 -> Is/1
  Ipv/1 -> Product4/2

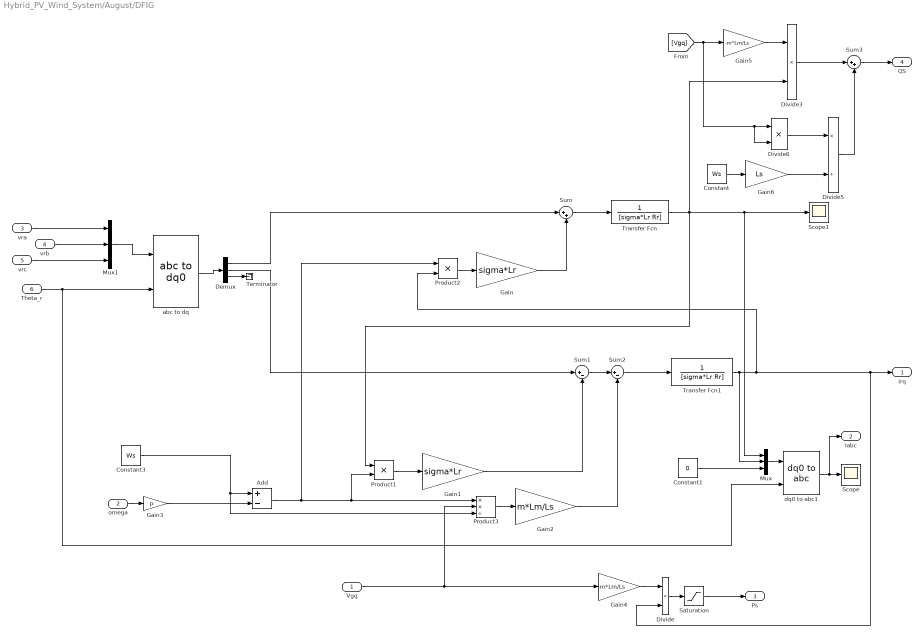
== system Hybrid_PV_Wind_System/August/DFIG  ==
  Vgq : Inport
  omega : Inport  Port=2
  vra : Inport  Port=3
  vrb : Inport  Port=4
  vrc : Inport  Port=5
  Theta_r : Inport  Port=6
  Add : Sum  Inputs=+-
  Constant : Constant  Value=Ws
  Constant1 : Constant  Value=0
  Constant3 : Constant  Value=Ws
  Demux : Demux  Outputs=3
  Divide : Product  Inputs=**
  Divide3 : Product  Inputs=**
  Divide5 : Product  Inputs=*/
  Divide6 : Product  Inputs=**
  Gain : Gain  Gain=sigma*Lr
  Gain1 : Gain  Gain=sigma*Lr
  Gain2 : Gain  Gain=m*Lm/Ls
  Gain3 : Gain  Gain=p
  Gain4 : Gain  Gain=m*Lm/Ls
  Gain5 : Gain  Gain=-m*Lm/Ls
  Gain6 : Gain  Gain=Ls
  Mux : Mux  Inputs=3
  Mux1 : Mux  Inputs=3
  Product1 : Product
  Product2 : Product
  Product3 : Product  Inputs=**/
  Saturation : Saturate  UpperLimit=0  LowerLimit=-3e6
  Scope : Scope
  Scope1 : Scope
  Sum : Sum  Inputs=|++
  Sum1 : Sum  Inputs=|+-
  Sum2 : Sum  Inputs=|+-
  Sum3 : Sum  Inputs=|++
  Terminator : Terminator
  Transfer Fcn : TransferFcn  Denominator=[sigma*Lr Rr]
  Transfer Fcn1 : TransferFcn  Denominator=[sigma*Lr Rr]
  abc to dq : powerlib_meascontrol/Transformations/abc to dq0  Alignment=90 degrees behind phase A axis
  dq0 to abc1 : powerlib_meascontrol/Transformations/dq0 to abc  Alignment=90 degrees behind phase A axis
  irq : Outport
  Iabc : Outport  Port=2
  Ps : Outport  Port=3
  QS : Outport  Port=4
  wires:
  Transfer Fcn/1 -> Scope1/1, Mux/1, Divide3/2, Product1/1
  Sum/1 -> Transfer Fcn/1
  Demux/2 -> Sum1/1
  Demux/1 -> Sum/1
  Product2/1 -> Gain/1
  Gain/1 -> Sum/2
  Constant3/1 -> Product3/3, Add/1
  Product1/1 -> Gain1/1
  Product3/1 -> Gain2/1
  Sum1/1 -> Sum2/1
  Gain1/1 -> Sum1/2
  Gain2/1 -> Sum2/2
  Sum2/1 -> Transfer Fcn1/1
  Add/1 -> Product2/1, Product1/2, Product3/1
  omega/1 -> Gain3/1
  Gain3/1 -> Add/2
  Constant1/1 -> Mux/3
  Mux/1 -> dq0 to abc1/1
  dq0 to abc1/1 -> Iabc/1, Scope/1
  abc to dq/1 -> Demux/1
  Demux/3 -> Terminator/1
  Mux1/1 -> abc to dq/1
  vra/1 -> Mux1/1
  vrb/1 -> Mux1/2
  vrc/1 -> Mux1/3
  Theta_r/1 -> dq0 to abc1/2, abc to dq/2
  Transfer Fcn1/1 -> irq/1, Divide/2, Product2/2, Mux/2
  Divide/1 -> Saturation/1
  Gain4/1 -> Divide/1
  Gain5/1 -> Divide3/1
  Divide3/1 -> Sum3/1
  Sum3/1 -> QS/1
  [Vgq] -> Divide6/2, Divide6/1, Gain5/1
  Divide6/1 -> Divide5/1
  Gain6/1 -> Divide5/2
  Constant/1 -> Gain6/1
  Divide5/1 -> Sum3/2
  Vgq/1 -> Product3/2, Gain4/1
  Saturation/1 -> Ps/1

== system Hybrid_PV_Wind_System/August/DHI8 ==
  Demux : Demux  Tag=STV Demux  Outputs=1
      settings: DisplayOption=none
  FromWs : FromWorkspace  Tag=STV FromWs  VariableName=tuvar
      SigBuilderData=|
      | common.afterFinalStr = 'Extrapolate'
      | common.sampleTime = 0
      | dataSet.timeRange = [0 750]
      | dataSet.name = 'Group 1'
      | sbobj.Groups.Name = 'Group 1'
      | sbobj.Groups.Signals.Name = 'Signal 1'
      | sbobj.Groups.Signals.XData = [0 1 2 3 4 5 6 7 8 9 10 11 ... (744 elements, 1x744)]
      | sbobj.Groups.Signals.YData = [0 0 0 0 0 0 6 79 95 102 130 160 ... (744 elements, 1x744)]
      | sbobj.Groups.TimeRange = [0 750]
  Signal 1 : Outport  Tag=STV Outport
  wires:
  FromWs/1 -> Demux/1
  Demux/1 -> Signal 1/1

== system Hybrid_PV_Wind_System/August/DNI8 ==
  Demux : Demux  Tag=STV Demux  Outputs=1
      settings: DisplayOption=none
  FromWs : FromWorkspace  Tag=STV FromWs  VariableName=tuvar
      SigBuilderData=|
      | common.afterFinalStr = 'Extrapolate'
      | common.sampleTime = 0
      | dataSet.timeRange = [0 750]
      | dataSet.name = 'Group 1'
      | sbobj.Groups.Name = 'Group 1'
      | sbobj.Groups.Signals.Name = 'Signal 1'
      | sbobj.Groups.Signals.XData = [0 1 2 3 4 5 6 7 8 9 10 11 ... (744 elements, 1x744)]
      | sbobj.Groups.Signals.YData = [0 0 0 0 0 0 0 325 691 784 826 833 ... (744 elements, 1x744)]
      | sbobj.Groups.TimeRange = [0 750]
  Signal 1 : Outport  Tag=STV Outport
  wires:
  FromWs/1 -> Demux/1
  Demux/1 -> Signal 1/1

== system Hybrid_PV_Wind_System/August/GHI8 ==
  Demux : Demux  Tag=STV Demux  Outputs=1
      settings: DisplayOption=none
  FromWs : FromWorkspace  Tag=STV FromWs  VariableName=tuvar
      SigBuilderData=|
      | common.afterFinalStr = 'Extrapolate'
      | common.sampleTime = 0
      | dataSet.timeRange = [0 750]
      | dataSet.name = 'Group 1'
      | sbobj.Groups.Name = 'Group 1'
      | sbobj.Groups.Signals.Name = 'Signal 1'
      | sbobj.Groups.Signals.XData = [0 1 2 3 4 5 6 7 8 9 10 11 ... (744 elements, 1x744)]
      | sbobj.Groups.Signals.YData = [0 0 0 0 0 0 6 171 389 604 790 921 ... (744 elements, 1x744)]
      | sbobj.Groups.TimeRange = [0 750]
  Signal 1 : Outport  Tag=STV Outport
  wires:
  Demux/1 -> Signal 1/1
  FromWs/1 -> Demux/1

== system Hybrid_PV_Wind_System/August/Gm1 ==
  Hour : Inport
  DNI : Inport  Port=2
  DHI : Inport  Port=3
  GHI : Inport  Port=4
  Irradiation : MATLAB Function  TreatAsAtomicUnit=on
  G_m : Outport
  wires:
  DHI/1 -> Irradiation/3(o)
  Irradiation/1(y) -> G_m/1
  DNI/1 -> Irradiation/2(k)
  GHI/1 -> Irradiation/4(p)
  Hour/1 -> Irradiation/1(i)

== system Hybrid_PV_Wind_System/August/Grid 1 ==
  Add1 : Sum  Inputs=-+
  Clock : Clock
  Constant : Constant  Value=2*pi
  Constant1 : Constant  Value=pi/2
  Demux : Demux  Outputs=3
  Gain : Gain  Gain=2*pi*50
  Manual Switch : ManualSwitch
  Math Function : Math  Operator=mod  SaturateOnIntegerOverflow=on
  Mux1 : Mux  Inputs=2
  PLL (3ph) : powerlib_meascontrol/PLL/PLL (3ph)  Fmin=45  Par_Init=[0, 50]  ParK=[180, 3200, 1]  TcD=1e-4  MaxRateChangeFreq=12  FilterCutOffFreq=25  Ts=0  AGC=on
  Scope : Scope
  Scope1 : Scope
  Terminator1 : Terminator
  Terminator2 : Terminator
  abc to dq1 : powerlib_meascontrol/Transformations/abc to dq0  Alignment=90 degrees behind phase A axis
  source : Sin  Amplitude=690*sqrt(2)/sqrt(3)  Frequency=2*pi*50  Phase=[0 -2*pi/3 2*pi/3]  SampleTime=0
  Vgd : Outport
  wt : Outport  Port=2
  Vgq : Outport  Port=3
  wires:
  abc to dq1/1 -> Demux/1
  source/1 -> abc to dq1/1, PLL (3ph)/1
  Demux/2 -> Mux1/2, Vgq/1
  Demux/3 -> Terminator1/1
  PLL (3ph)/1 -> Terminator2/1
  Clock/1 -> Gain/1
  PLL (3ph)/2 -> Manual Switch/1
  Gain/1 -> Math Function/1
  Constant/1 -> Math Function/2
  Math Function/1 -> Manual Switch/2
  Add1/1 -> abc to dq1/2, wt/1
  Mux1/1 -> Scope/1
  Constant1/1 -> Add1/1
  Manual Switch/1 -> Add1/2
  Demux/1 -> Mux1/1, Scope1/1, Vgd/1

== system Hybrid_PV_Wind_System/August/Hours8 ==
  Demux : Demux  Tag=STV Demux  Outputs=1
      settings: DisplayOption=none
  FromWs : FromWorkspace  Tag=STV FromWs  VariableName=tuvar
      SigBuilderData=|
      | common.afterFinalStr = 'Extrapolate'
      | common.sampleTime = 0
      | dataSet.timeRange = [0 750]
      | dataSet.name = 'Group 1'
      | sbobj.Groups.Name = 'Group 1'
      | sbobj.Groups.Signals.Name = 'Signal 1'
      | sbobj.Groups.Signals.XData = [0 1 2 3 4 5 6 7 8 9 10 11 ... (745 elements, 1x745)]
      | sbobj.Groups.Signals.YData = [0 1 2 3 4 5 6 7 8 9 10 11 ... (745 elements, 1x745)]
      | sbobj.Groups.TimeRange = [0 750]
  Signal 1 : Outport  Tag=STV Outport
  wires:
  Demux/1 -> Signal 1/1
  FromWs/1 -> Demux/1

== system Hybrid_PV_Wind_System/August/Hub height spped ==
  V : Inport
  Constant : Constant  Value=Z_hub
  Constant5 : Constant  Value=Z_data
  Constant6 : Constant  Value=Z_0
  Divide : Product  Inputs=*/
  Divide1 : Product  Inputs=*/
  Divide2 : Product  Inputs=*/
  Math Function : Math  Operator=log  SaturateOnIntegerOverflow=on
  Math Function1 : Math  Operator=log  SaturateOnIntegerOverflow=on
  Product : Product
  V_hub : Outport
  wires:
  Divide1/1 -> Math Function/1
  Divide2/1 -> Product/1
  Constant6/1 -> Divide1/2, Divide/2
  Constant5/1 -> Divide1/1
  Divide/1 -> Math Function1/1
  Constant/1 -> Divide/1
  Math Function1/1 -> Divide2/1
  Math Function/1 -> Divide2/2
  Product/1 -> V_hub/1
  V/1 -> Product/2

== system Hybrid_PV_Wind_System/August/MPPT1 ==
  I : Inport
  V : Inport  Port=2
  CI : MATLAB Function  TreatAsAtomicUnit=on
  DP : Sum  Inputs=+-
  DV1 : Sum  Inputs=+-
  Memory2 : Memory
  Pk : Product  Inputs=**
  Pk-1 : Memory  InitialCondition=-0.1
  Unit Delay1 : UnitDelay  SampleTime=1e-4  HasFrameUpgradeWarning=on
  Vmpp : Outport
  wires:
  DP/1 -> CI/2(DP)
  DV1/1 -> CI/1(DV)
  CI/1(d) -> Unit Delay1/1
  Pk-1/1 -> DP/2
  Pk/1 -> Pk-1/1, DP/1
  V/1 -> Pk/1, Memory2/1, DV1/1
  Memory2/1 -> DV1/2
  I/1 -> Pk/2
  Unit Delay1/1 -> Vmpp/1

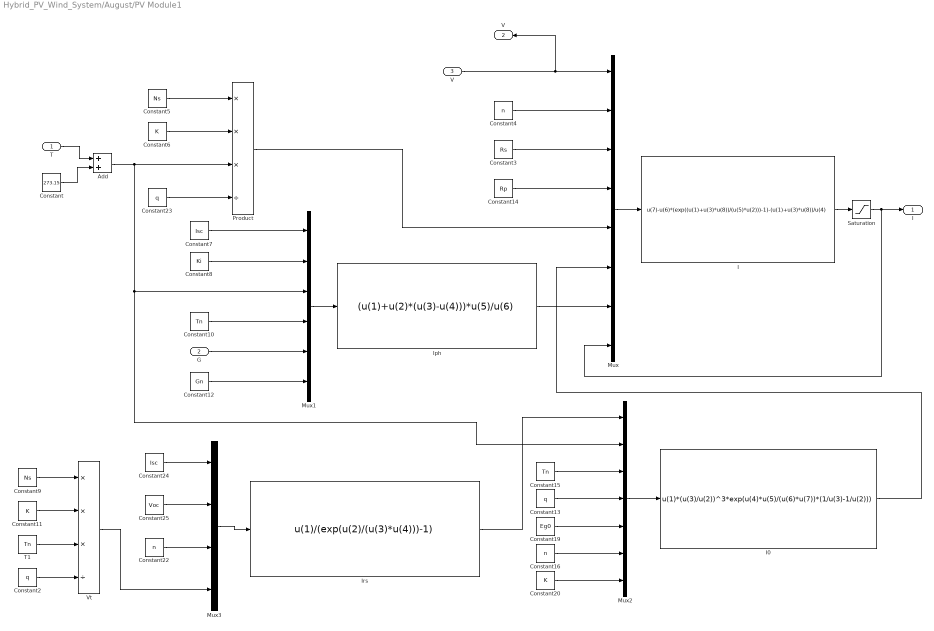
== system Hybrid_PV_Wind_System/August/PV Module1 ==
  T : Inport
  G : Inport  Port=2
  "V " : Inport  Port=3
  Add : Sum
  Constant : Constant  Value=273.15
  Constant10 : Constant  Value=Tn
  Constant11 : Constant  Value=K
  Constant12 : Constant  Value=Gn
  Constant13 : Constant  Value=q
  Constant14 : Constant  Value=Rp
  Constant15 : Constant  Value=Tn
  Constant16 : Constant  Value=n
  Constant19 : Constant  Value=Eg0
  Constant2 : Constant  Value=q
  Constant20 : Constant  Value=K
  Constant22 : Constant  Value=n
  Constant23 : Constant  Value=q
  Constant24 : Constant  Value=Isc
  Constant25 : Constant  Value=Voc
  Constant3 : Constant  Value=Rs
  Constant4 : Constant  Value=n
  Constant5 : Constant  Value=Ns
  Constant6 : Constant  Value=K
  Constant7 : Constant  Value=Isc
  Constant8 : Constant  Value=Ki
  Constant9 : Constant  Value=Ns
  "I " : Fcn  Expr=u(7)-u(6)*(exp((u(1)+u(3)*u(8))/(u(5)*u(2)))-1)-(u(1)+u(3)*u(8))/u(4)
  I0 : Fcn  Expr=u(1)*(u(3)/u(2))^3*exp(u(4)*u(5)/(u(6)*u(7))*(1/u(3)-1/u(2)))
  Iph : Fcn  Expr=(u(1)+u(2)*(u(3)-u(4)))*u(5)/u(6)
  Irs : Fcn  Expr=u(1)/(exp(u(2)/(u(3)*u(4)))-1)
  Mux : Mux  Inputs=8
  Mux1 : Mux  Inputs=6
  Mux2 : Mux  Inputs=7
  Mux3 : Mux
  Product : Product  Inputs=***/
  Saturation : Saturate  UpperLimit=10  LowerLimit=0
  T1 : Constant  Value=Tn
  Vt : Product  Inputs=***/
  I : Outport
  V : Outport  Port=2
  wires:
  Constant5/1 -> Product/1
  Constant20/1 -> Mux2/7
  Constant4/1 -> Mux/2
  Constant3/1 -> Mux/3
  Product/1 -> Mux/5
  "V "/1 -> V/1, Mux/1
  Mux/1 -> "I "/1
  Constant14/1 -> Mux/4
  Mux1/1 -> Iph/1
  Constant8/1 -> Mux1/2
  Constant10/1 -> Mux1/4
  G/1 -> Mux1/5
  Iph/1 -> Mux/7
  Constant7/1 -> Mux1/1
  Constant12/1 -> Mux1/6
  Constant15/1 -> Mux2/3
  Mux2/1 -> I0/1
  Constant13/1 -> Mux2/4
  Constant19/1 -> Mux2/5
  I0/1 -> Mux/6
  Constant16/1 -> Mux2/6
  Add/1 -> Mux2/2, Mux1/3, Product/3
  Mux3/1 -> Irs/1
  Constant24/1 -> Mux3/1
  Constant22/1 -> Mux3/3
  Constant25/1 -> Mux3/2
  Irs/1 -> Mux2/1
  Constant2/1 -> Vt/4
  T1/1 -> Vt/3
  Constant9/1 -> Vt/1
  Constant11/1 -> Vt/2
  Vt/1 -> Mux3/4
  Constant6/1 -> Product/2
  Constant23/1 -> Product/4
  "I "/1 -> Saturation/1
  Constant/1 -> Add/2
  T/1 -> Add/1
  Saturation/1 -> I/1, Mux/8

== system Hybrid_PV_Wind_System/August/PWM ==
  Vrd_ : Inport
  Vrq_ : Inport  Port=2
  theta_r : Inport  Port=3
  Constant : Constant  Value=0
  Constant1 : Constant
  Constant2 : Constant  Value=-1
  Demux1 : Demux  Outputs=3
  Mux2 : Mux  Inputs=3
  Relational Operator : RelationalOperator  OutDataTypeStr=boolean  RndMeth=Nearest
  Relational Operator1 : RelationalOperator  OutDataTypeStr=boolean  RndMeth=Nearest
  Relational Operator2 : RelationalOperator  OutDataTypeStr=boolean  RndMeth=Nearest
  Repeating Sequence : simulink/Sources/Repeating Sequence  rep_seq_t=[0 1/40000 1/20000 3/40000 1/10000]  rep_seq_y="[0 600  0 -600 0]"
  Scope3 : Scope
  Scope5 : Scope
  Scope6 : Scope
  Switch : Switch  Criteria=u2 > Threshold
  Switch1 : Switch  Criteria=u2 > Threshold
  Switch2 : Switch  Criteria=u2 > Threshold
  dq0 to abc1 : powerlib_meascontrol/Transformations/dq0 to abc  Alignment=90 degrees behind phase A axis
  PWMa : Outport
  PWMb : Outport  Port=2
  PWMc : Outport  Port=3
  wires:
  Constant/1 -> Mux2/3
  Switch2/1 -> PWMc/1
  Switch1/1 -> PWMb/1
  Switch/1 -> PWMa/1
  Demux1/2 -> Relational Operator1/2
  Demux1/3 -> Relational Operator2/2
  Demux1/1 -> Relational Operator/2
  Repeating Sequence/1 -> Scope6/1, Relational Operator2/1, Relational Operator1/1, Relational Operator/1
  Constant2/1 -> Switch/3, Switch1/3, Switch2/3
  Mux2/1 -> dq0 to abc1/1, Scope5/1
  Relational Operator2/1 -> Switch2/2
  Vrd_/1 -> Mux2/1
  Constant1/1 -> Switch1/1, Switch2/1, Switch/1
  Relational Operator/1 -> Switch/2
  Relational Operator1/1 -> Switch1/2
  Vrq_/1 -> Mux2/2
  theta_r/1 -> dq0 to abc1/2
  dq0 to abc1/1 -> Demux1/1, Scope3/1

== system Hybrid_PV_Wind_System/August/RL Filtre ==
  note: RL filter
  note: DC Bus
  note: Id
  note: Iq
  abc : Inport
  Vgd : Inport  Port=2
  wt : Inport  Port=3
  Vgq : Inport  Port=4
  Irq : Inport  Port=5
  Add : Sum
  Demux1 : Demux  Outputs=3
  Gain : Gain  Gain=L*Ws
  Gain1 : Gain  Gain=1/c
  Gain2 : Gain  Gain=L*Ws
  Integrator : Integrator  UpperSaturationLimit=2000  LowerSaturationLimit=-2000
  Sum : Sum  Inputs=-+-
  Sum2 : Sum  Inputs=-++
  Terminator : Terminator
  Transfer Fcn : TransferFcn  Denominator=[L R]
  Transfer Fcn1 : TransferFcn  Denominator=[L R]
  abc to dq1 : powerlib_meascontrol/Transformations/abc to dq0  Alignment=90 degrees behind phase A axis
  Id : Outport
  Iq : Outport  Port=2
  Vdc : Outport  Port=3
  wires:
  Transfer Fcn1/1 -> Iq/1, Add/1, Gain/1
  abc to dq1/1 -> Demux1/1
  Demux1/3 -> Terminator/1
  abc/1 -> abc to dq1/1
  wt/1 -> abc to dq1/2
  Sum/1 -> Transfer Fcn/1
  Sum2/1 -> Transfer Fcn1/1
  Gain/1 -> Sum/3
  Gain2/1 -> Sum2/3
  Add/1 -> Gain1/1
  Gain1/1 -> Integrator/1
  Transfer Fcn/1 -> Id/1, Gain2/1
  Demux1/2 -> Sum2/2
  Demux1/1 -> Sum/2
  Irq/1 -> Add/2
  Vgq/1 -> Sum2/1
  Vgd/1 -> Sum/1
  Integrator/1 -> Vdc/1

== system Hybrid_PV_Wind_System/August/RL Filtre1 ==
  abc : Inport
  Vgq : Inport  Port=2
  wt : Inport  Port=3
  Demux1 : Demux  Outputs=3
  Gain : Gain  Gain=L*Ws/Vgq
  Gain2 : Gain  Gain=L*Ws/Vgq
  Sum : Sum  Inputs=-++
  Sum1 : Sum  Inputs=|+-
  Terminator : Terminator
  Transfer Fcn : TransferFcn  Denominator="[L1/Vgq  R1/Vgq ]"
  Transfer Fcn1 : TransferFcn  Denominator="[L1/Vgq  R1/Vgq ]"
  abc to dq : powerlib_meascontrol/Transformations/abc to dq0  Alignment=90 degrees behind phase A axis
  "Q " : Outport
  P : Outport  Port=2
  wires:
  Transfer Fcn/1 -> "Q "/1, Gain2/1
  Demux1/1 -> Sum1/1
  Demux1/2 -> Sum/2
  abc to dq/1 -> Demux1/1
  Demux1/3 -> Terminator/1
  abc/1 -> abc to dq/1
  wt/1 -> abc to dq/2
  Vgq/1 -> Sum/1
  Gain2/1 -> Sum/3
  Gain/1 -> Sum1/2
  Sum1/1 -> Transfer Fcn/1
  Sum/1 -> Transfer Fcn1/1
  Transfer Fcn1/1 -> P/1, Gain/1

== system Hybrid_PV_Wind_System/August/RSC ==
  Vdc : Inport
  pwma : Inport  Port=2
  pwmb : Inport  Port=3
  pwmc : Inport  Port=4
  Fcn : Fcn  Expr=u(1)/6*(2*u(2)-u(3)-u(4))
  Fcn1 : Fcn  Expr=u(1)/6*(-u(2)+2*u(3)-u(4))
  Fcn2 : Fcn  Expr=u(1)/6*(-u(2)-u(3)+2*u(4))
  Mux : Mux
  Mux1 : Mux  Inputs=3
  Scope4 : Scope
  Via : Outport
  Vib : Outport  Port=2
  Vic : Outport  Port=3
  wires:
  Vdc/1 -> Mux/1
  Mux/1 -> Fcn2/1, Fcn1/1, Fcn/1
  pwma/1 -> Mux/2
  pwmb/1 -> Mux/3
  pwmc/1 -> Mux/4
  Fcn/1 -> Mux1/1, Via/1
  Fcn1/1 -> Vib/1, Mux1/2
  Fcn2/1 -> Vic/1, Mux1/3
  Mux1/1 -> Scope4/1

== system Hybrid_PV_Wind_System/August/T cell 1 ==
  T : Inport
  G : Inport  Port=2
  Add : Sum  Inputs=+-
  Add1 : Sum
  Constant2 : Constant  Value=NOCT
  Constant4 : Constant  Value=20
  Gain1 : Gain  Gain=1/80
  Gain2 : Gain  Gain=1/10
  Product3 : Product
  Tc : Outport
  wires:
  Constant2/1 -> Add/1
  Product3/1 -> Gain1/1
  Constant4/1 -> Add/2
  Add/1 -> Product3/1
  Gain2/1 -> Product3/2
  Gain1/1 -> Add1/1
  G/1 -> Gain2/1
  T/1 -> Add1/2
  Add1/1 -> Tc/1
